simulink model "localReroute_fsm"  (R2022a)
settings: Solver=VariableStepAuto  StartTime=0.0  StopTime=10.0  RelTol=1e-3
settings Model: Creator=Nate  LastModifiedBy=Nate
settings DebuggingCC: UnconnectedInputMsg=warning  UnconnectedOutputMsg=warning  UnconnectedLineMsg=warning
settings RTWCC: DLArmComputeVersion=19.05

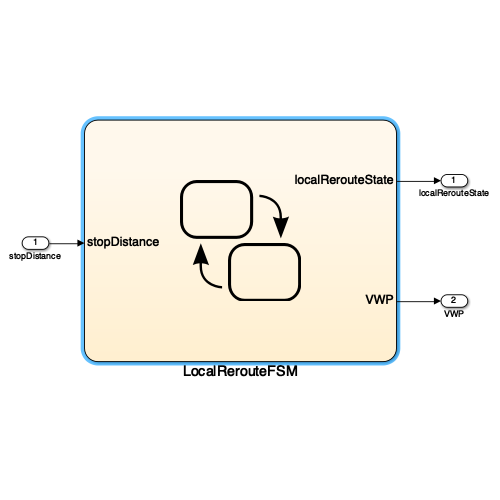
[thumbnail: Simulink's stored preview of the top-level diagram]
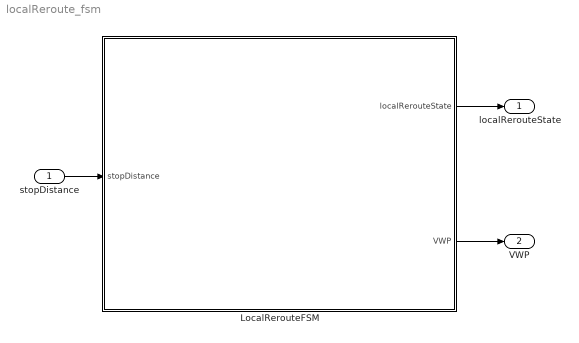
== system localReroute_fsm ==
  stopDistance : Inport
  LocalRerouteFSM : Stateflow chart  TreatAsAtomicUnit=on
  localRerouteState : Outport
  VWP : Outport  Port=2
  wires:
  stopDistance/1 -> LocalRerouteFSM/1(stopDistance)
  LocalRerouteFSM/1(localRerouteState) -> localRerouteState/1
  LocalRerouteFSM/2(VWP) -> VWP/1

== stateflow chart localReroute_fsm/LocalRerouteFSM ==
  state localReroute [group]
    state wait_for_localReroute_enable
      en:  localRerouteState = 0;
    state slow_while_rerouting
      en: localRerouteState = 1
      du: newVWP = calculateLocalRoute()
      ex: turnSignalLightOn()
    (default) -> wait_for_localReroute_enable
    wait_for_localReroute_enable -> wait_for_localReroute_enable [order 2]
    slow_while_rerouting -> wait_for_localReroute_enable [order 1] : [LocalRerouteEnable == false || newVWP.length > 0]
        | { updateWaypoints(newVWP);
        |   SubMachineRunning = false;
        |   LocalRerouteEnable = false; }
    wait_for_localReroute_enable -> slow_while_rerouting [order 1] : [LocalRerouteEnable == true]
        | {VWP = updateVWP(VWP, stopDistance)}
    slow_while_rerouting -> slow_while_rerouting [order 2]
  data: SubMachineRunning data_store_memory; localRerouteState output; newVWP local; VWP output; LocalRerouteEnable data_store_memory; stopDistance input
